simulink model "W09_P1"  (R2024b)
settings: Solver=ode4  StartTime=0  StopTime=T_final  FixedStep=h  RelTol=1e-3
undefined symbols (not defined in the file or in its folder): a_i, beta_c, Delta, e_min, h, hand_over, k_neg, k_pos, k_w, kappa, Kd, Kd_x, Ki_u, Ki_x, Kp, Kp_u, Kp_x, mp, N_max, N_open, phi_i, rp, T_max, T_min, u_d, use_ilos, use_Kd, use_Ki_u, use_scale, use_ssa, use_vane, V_c, w0, w_i, wave_on, WP_E, WP_N, x0, X_max, y_pont, zeta_d, zeta_n
settings Model: Creator=admin  LastModifiedBy=admin
settings DataIOCC: ReturnWorkspaceOutputs=off

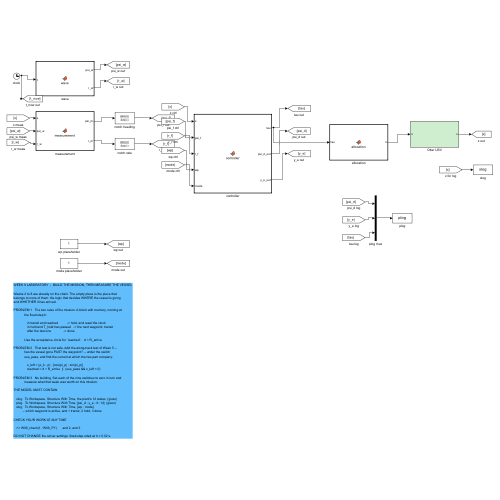
[thumbnail: Simulink's stored preview of the top-level diagram]
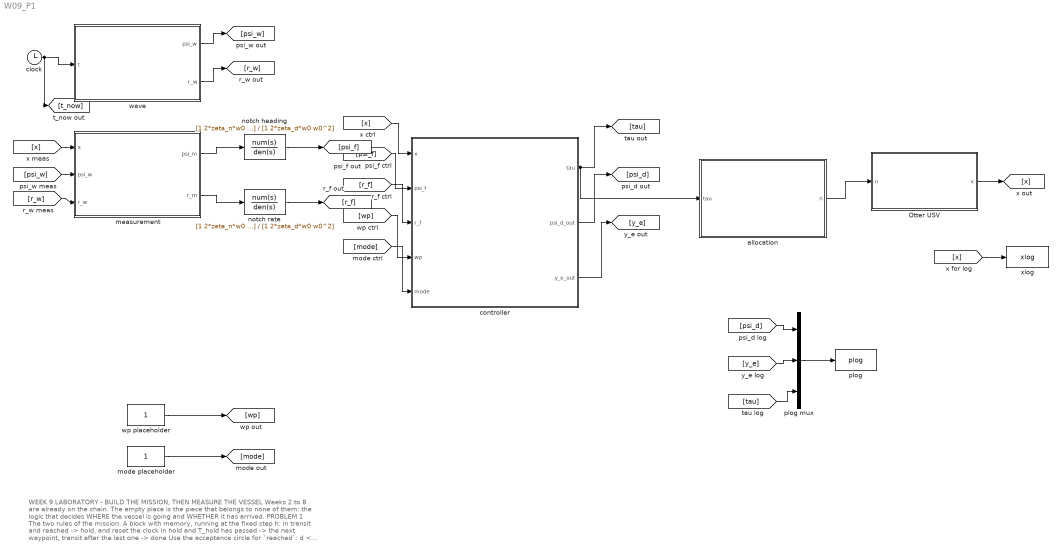
== system W09_P1 ==
  note: WEEK 9 LABORATORY  -  BUILD THE MISSION, THEN MEASURE THE VESSEL
      |
      | Weeks 2 to 8 are already on the chain. The empty place is the piece that
      | belongs to none of them: the logic that decides WHERE the vessel is going
      | and WHETHER it has arrived.
      |
      | PROBLEM 1   The two rules of the mission. A block with memory, running at
      |             the fixed step h:
      |
      |                in transit and reached          -> hold, and reset the clock
      |                in hold and T_hold has passed   -> the next waypoint, transit
      |                after the last one              -> done
      |
      |             Use the acceptance circle for `reached`:   d < R_arrive
      |
      | PROBLEM 2   That test is not safe. Add the along-track test of Week 5 --
      |             has the vessel gone PAST the waypoint? -- under the switch
      |             use_pass, and find the current at which the two part company:
      |
      |                x_left = (p_k - p) . [cos(pi_p) ; sin(pi_p)]
      |                reached = d < R_arrive  ||  (use_pass && x_left < 0)
      |
      | PROBLEM 3   No building. Set each of the nine switches to zero in turn and
      |             measure what that week was worth on this mission.
      |
      | THE MODEL MUST CONTAIN
      |
      |    xlog   To Workspace, Structure With Time, the plant's 12 states  (given)
      |    plog   To Workspace, Structure With Time, [psi_d ; y_e ; X ; N]  (given)
      |    slog   To Workspace, Structure With Time, [wp ; mode]
      |           -- which waypoint is active, and 1 transit, 2 hold, 3 done
      |
      | CHECK YOUR WORK AT ANY TIME
      |
      |    >> W09_check(1, 'W09_P1')      and 2, and 3
      |
      | DO NOT CHANGE the solver settings: fixed-step ode4 at h = 0.02 s.
  Otter USV : Subsystem
  allocation : MATLAB Function  TreatAsAtomicUnit=on
  clock : Clock
  controller : MATLAB Function  TreatAsAtomicUnit=on
  measurement : MATLAB Function  TreatAsAtomicUnit=on
  mode placeholder : Constant
  notch heading : TransferFcn  Numerator=[1 2*zeta_n*w0 w0^2]  Denominator=[1 2*zeta_d*w0 w0^2]
  notch rate : TransferFcn  Numerator=[1 2*zeta_n*w0 w0^2]  Denominator=[1 2*zeta_d*w0 w0^2]
  plog : ToWorkspace  VariableName=plog  SaveFormat=Structure With Time  SampleTime=-1
  plog mux : Mux  Inputs=3
  wave : MATLAB Function  TreatAsAtomicUnit=on
  wp placeholder : Constant
  xlog : ToWorkspace  VariableName=xlog  SaveFormat=Structure With Time  SampleTime=-1
  wires:
  clock/1 -> wave/1(t), [t_now]
  wave/1(psi_w) -> [psi_w]
  wave/2(r_w) -> [r_w]
  [x] -> measurement/1(x)
  [psi_w] -> measurement/2(psi_w)
  [r_w] -> measurement/3(r_w)
  measurement/1(psi_m) -> notch heading/1
  notch heading/1 -> [psi_f]
  measurement/2(r_m) -> notch rate/1
  notch rate/1 -> [r_f]
  [x] -> controller/1(x)
  [psi_f] -> controller/2(psi_f)
  [r_f] -> controller/3(r_f)
  [wp] -> controller/4(wp)
  [mode] -> controller/5(mode)
  controller/1(tau) -> [tau], allocation/1(tau)
  controller/2(psi_d_out) -> [psi_d]
  controller/3(y_e_out) -> [y_e]
  allocation/1(n) -> Otter USV/1(n)
  Otter USV/1(x) -> [x]
  [x] -> xlog/1
  [psi_d] -> plog mux/1
  [y_e] -> plog mux/2
  [tau] -> plog mux/3
  plog mux/1 -> plog/1
  wp placeholder/1 -> [wp]
  mode placeholder/1 -> [mode]

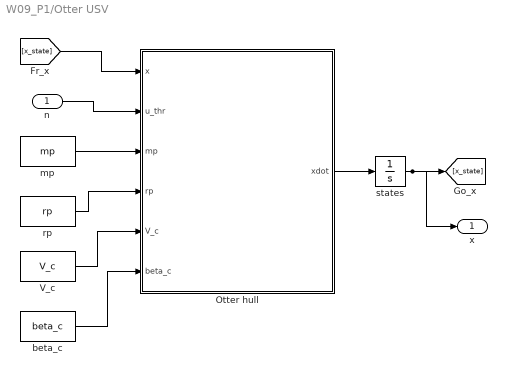
== system W09_P1/Otter USV ==
  n : Inport
  Otter hull : MATLAB Function  TreatAsAtomicUnit=on
  V_c : Constant  Value=V_c
  beta_c : Constant  Value=beta_c
  mp : Constant  Value=mp
  rp : Constant  Value=rp
  states : Integrator  InitialCondition=x0
  x : Outport
  wires:
  mp/1 -> Otter hull/3(mp)
  [x_state] -> Otter hull/1(x)
  beta_c/1 -> Otter hull/6(beta_c)
  n/1 -> Otter hull/2(u_thr)
  rp/1 -> Otter hull/4(rp)
  V_c/1 -> Otter hull/5(V_c)
  Otter hull/1(xdot) -> states/1
  states/1 -> [x_state], x/1

== matlab function W09_P1/Otter USV/Otter hull ==
  data: x input; xdot output double size=[12 1]; u_thr input; mp input; rp input; V_c input; beta_c input
function xdot = otter_hull(x, u_thr, mp, rp, V_c, beta_c)
% Fossen's otter.m, called unchanged from Tools/MSS/VESSELS.
%
%   x       12 states, fed back from the integrator
%   u_thr   propeller shaft speeds [rad/s]
%
% otter.m is not written for code generation, so the call is extrinsic and
% xdot has to be pre-sized for Simulink to know the output width.
coder.extrinsic('otter');

xdot = zeros(12,1);
xdot = otter(x, u_thr, mp, rp, V_c, beta_c);
end

== matlab function W09_P1/measurement ==
  data: x input; psi_m output double size=[1 1]; psi_w input; r_w input; r_m output
function [psi_m, r_m] = measurement(x, psi_w, r_w)
%#codegen
%  제어기가 보는 것 = 배가 하는 것 + 1차 파랑 (7주차 §7-2)
psi_m = x(12)*180/pi + psi_w;
r_m   = x(6)*180/pi  + r_w;

== matlab function W09_P1/wave ==
  data: t input; psi_w output double size=[1 1]; r_w output; w_i parameter; a_i parameter; phi_i parameter; k_w parameter; wave_on parameter
function [psi_w, r_w] = wave(t, w_i, a_i, phi_i, k_w, wave_on)
%#codegen
%  7주차의 바다 그대로 / the sea of Week 7, unchanged
psi_w = 0;  r_w = 0;
if wave_on ~= 0
    for i = 1:numel(w_i)
        psi_w = psi_w + k_w*a_i(i)*sin(w_i(i)*t + phi_i(i));
        r_w   = r_w   + k_w*a_i(i)*w_i(i)*cos(w_i(i)*t + phi_i(i));
    end
end

== matlab function W09_P1/controller ==
  settings: updateMethod=DISCRETE  sampleTime=h
  data: x input; tau output double size=[2 1]; psi_f input; r_f input; wp input; mode input; psi_d_out output; y_e_out output; WP_N parameter; WP_E parameter; Delta parameter; kappa parameter; u_d parameter; Kp_u parameter; Ki_u parameter; Kp parameter; Kd parameter; Kp_x parameter; Ki_x parameter; Kd_x parameter; e_min parameter; X_max parameter; N_max parameter; N_open parameter; use_Ki_u parameter; use_ssa parameter; use_Kd parameter; use_ilos parameter; use_scale parameter; use_vane parameter; hand_over parameter; h parameter
function [tau, psi_d_out, y_e_out] = controller(x, psi_f, r_f, wp, mode, WP_N, WP_E, Delta, kappa, u_d, Kp_u, Ki_u, Kp, Kd, Kp_x, Ki_x, Kd_x, e_min, X_max, N_max, N_open, use_Ki_u, use_ssa, use_Kd, use_ilos, use_scale, use_vane, hand_over, h)
%#codegen
%  여덟 주차가 한 블록에. 모드에 따라 어느 줄이 도는지가 달라질 뿐이다.
%  Eight weeks in one block; the mode decides which lines run.
psi = x(12);  u = x(1);  v = x(2);
psi_m = psi_f*pi/180;  r_m = r_f*pi/180;      % 노치를 지난 계측 (7주차)
k = wp;  y_e = 0;
persistent I_u y_int In Ie psi_last
if isempty(I_u), I_u = 0; y_int = 0; In = 0; Ie = 0; psi_last = psi; end
if mode == 1
    %  ── 이동 / transit ────────────────────────────────────────────────
    if k > 1, N0 = WP_N(k-1);  E0 = WP_E(k-1);  else, N0 = 0;  E0 = 0;  end
    pi_p = atan2(WP_E(k) - E0, WP_N(k) - N0);
    y_e  = -(x(7) - N0)*sin(pi_p) + (x(8) - E0)*cos(pi_p);
    if use_ilos ~= 0
        psi_d = pi_p - atan((y_e + kappa*y_int)/Delta);
        y_int = y_int + h*Delta*y_e/(Delta^2 + (y_e + kappa*y_int)^2);
    else
        psi_d = pi_p - atan(y_e/Delta);
    end
    eu = u_d - u;
    X  = Kp_u*eu + I_u;
    X  = min(max(X, -X_max), X_max);
    if use_Ki_u ~= 0 && abs(X) < X_max - 1e-9, I_u = I_u + h*Ki_u*eu; end
    if hand_over ~= 0, In = 0;  Ie = 0; end
    psi_last = psi_d;
else
    %  ── 유지 / hold ──────────────────────────────────────────────────
    e_n = WP_N(k) - x(7);  e_e = WP_E(k) - x(8);
    v_n = u*cos(psi) - v*sin(psi);  v_e = u*sin(psi) + v*cos(psi);
    f_n = Kp_x*e_n + In - Kd_x*v_n;
    f_e = Kp_x*e_e + Ie - Kd_x*v_e;
    if use_vane ~= 0
        if hypot(f_n, f_e) > e_min, psi_last = atan2(f_e, f_n); end
        psi_d = psi_last;
    else
        psi_d = psi_last;
    end
    X = f_n*cos(psi) + f_e*sin(psi);
    X = min(max(X, -X_max), X_max);
    if abs(X) < X_max - 1e-9
        In = In + h*Ki_x*e_n;  Ie = Ie + h*Ki_x*e_e;
    end
    I_u = 0;
end
%  ── 4주차: 선수각 / the heading loop ─────────────────────────────────
if use_ssa ~= 0
    ee = atan2(sin(psi_d - psi_m), cos(psi_d - psi_m));
else
    ee = psi_d - psi_m;
end
N  = Kp*ee;
if use_Kd ~= 0, N = N - Kd*r_m; end
N_lim = N_max;
if use_scale == 0, N_lim = N_open; end
N  = min(max(N, -N_lim), N_lim);
if mode == 3, X = 0;  N = 0; end
tau = [X; N];  psi_d_out = psi_d*180/pi;  y_e_out = y_e;

== matlab function W09_P1/allocation ==
  data: tau input; n output double size=[2 1]; y_pont parameter; k_pos parameter; k_neg parameter; T_max parameter; T_min parameter; use_scale parameter
function n = allocation(tau, y_pont, k_pos, k_neg, T_max, T_min, use_scale)
%#codegen
%  6주차의 배분 / the allocation of Week 6
T1 = tau(1)/2 + tau(2)/(2*y_pont);
T2 = tau(1)/2 - tau(2)/(2*y_pont);
if use_scale ~= 0
    s = 1;
    if T1 > T_max, s = min(s, T_max/T1); end
    if T2 > T_max, s = min(s, T_max/T2); end
    if T1 < T_min, s = min(s, T_min/T1); end
    if T2 < T_min, s = min(s, T_min/T2); end
    T1 = s*T1;  T2 = s*T2;
else
    T1 = min(max(T1, T_min), T_max);
    T2 = min(max(T2, T_min), T_max);
end
k1 = k_pos;  if T1 < 0, k1 = k_neg; end
k2 = k_pos;  if T2 < 0, k2 = k_neg; end
n = [sign(T1)*sqrt(abs(T1)/k1); sign(T2)*sqrt(abs(T2)/k2)];
